simulink model "controlNoLinealModeloCompleto"  (R2023b)
settings: Solver=VariableStepAuto  StartTime=0.0  StopTime=10.0  RelTol=1e-3
values from neighbouring files (symbols this model uses):
  qc = robot.ikine(Tcart,q0,'mask',mask)    [TP_2.m]
libraries: roblocks x8
settings Model: Creator=nmestanza  LastModifiedBy=nmestanza

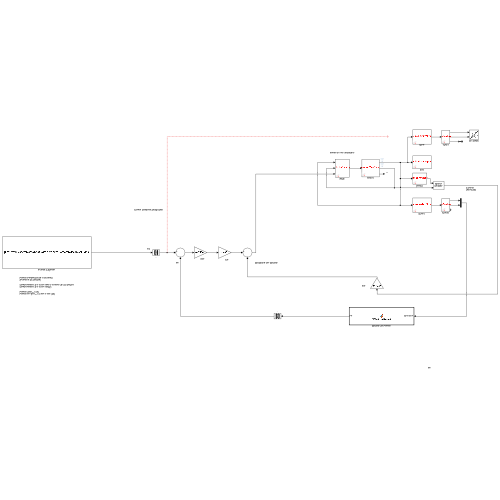
[thumbnail: Simulink's stored preview of the top-level diagram]
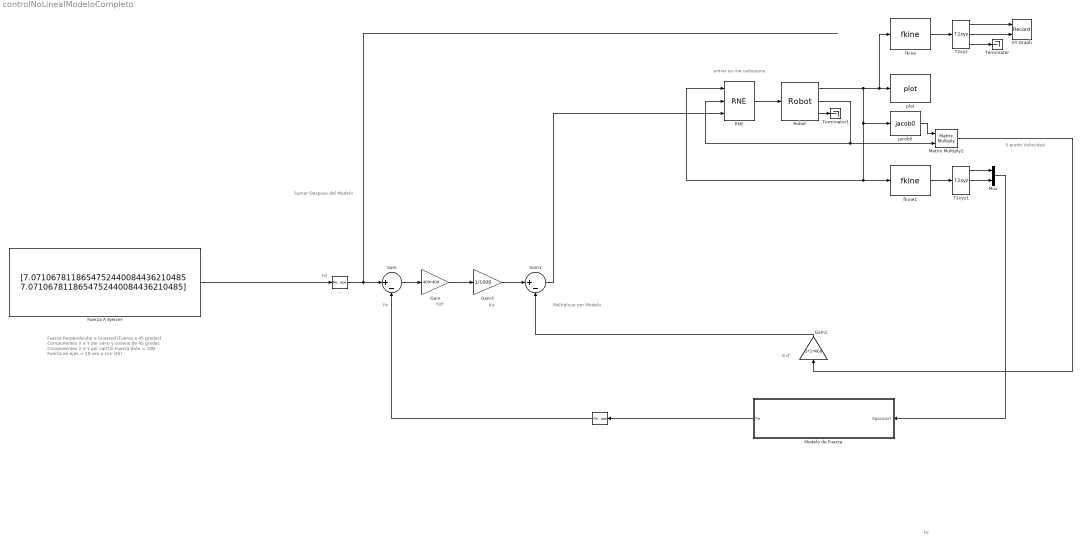
== system controlNoLinealModeloCompleto ==
  note: Multiplicar por Modelo
  note: Sumar Despues del Modelo
  note: X punto
      | Velocidad
  note: Fe
  note: Fe
  note: Kvf
  note: Kpf
  note: Fuerza Perpendicular a la pared
      | (Fuerza a 45 grados)
      |
      | Componentes X e Y por seno y coseno de 45 grados
      | Componentes X e Y por sqrt(2)
      |
      | Fuerza dato = 10N
      | Fuerza en ejes = 10.sen o cos (45)
  note: Ke
  note: Fd
  note: armar un rne cartesiano
  . : Reshape  OutputDimensionality=Column vector (2-D)
  .. : Reshape  OutputDimensionality=Column vector (2-D)
  Fuerza A Ejercer : Constant  Value=[7.0710678118654752440084436210485 7.0710678118654752440084436210485]
  Gain : Gain  Gain=400*400
  Gain1 : Gain  Gain=2*1*400
  Gain3 : Gain  Gain=1/1000
  Matrix Multiply2 : Product  Multiplication=Matrix(*)
  Modelo de Fuerza : MATLAB Function  TreatAsAtomicUnit=on
  Mux : Mux  Inputs=2
  RNE : roblocks/Arm/RNE  robot=robot  grav=[0 0 9.81]
  Robot : roblocks/Arm/Robot  robot=robot  q0=qc(1,:)
  Sum : Sum  Inputs=|+-
  Sum1 : Sum  Inputs=|+-
  T2xyz : roblocks/Toolbox/T2xyz
  T2xyz1 : roblocks/Toolbox/T2xyz
  Terminator : Terminator
  Terminator1 : Terminator
  XY Graph : Record  FileSettingsInternal="{\"entries\":[{\"content\":{\"excelSettings\":{\"content\":{},\"type\":\"Streamout.ExcelSettings\"}},\"type\":\"Streamout.FileSettingStorage\",\"uuid\":\"\"}],\"packageUris\":[\"http:\\/\\/schema.mathworks.com\\/mf0\\/streamout_blocks\\/R2020a\"],\"version\":\"1.0\"}"  Layout=[1 1]  SignalsInternal="{\"entries\":[{\"content\":{\"signals\":[{\"content\":{\"blockPath\":[],\"dimensions\":[1],\"domain\":\"\",\"lineColor\":\"#a2142f\",\"plots\":[1],\"port\":1,\"signalID\":32,\"signalName\":\"XY Graph:1\"},\"type\":\"RecordBlkView.Signal\",\"uuid\":\"\"},{\"content\":{\"blockPath\":[],\"dimensions\":[1],\"domain\":\"\",\"lineColor\":\"#139fff\",\"plots\":[1],\"port\":2,\"signalID\":35,\"signalName\":\"XY Graph:2\"},\"type\":\"RecordBlkView.Signal\",\"uuid\":\"\"}]},\"type\":\"RecordBlkView.InputSignals\",\"uuid\":\"\"}],\"packageUris\":[\"http:\\/\\/schema.mathworks.com\\/mf0\\/streamout_blocks\\/R2020a\"],\"version\":\"1.0\"}"  VisualizationBindings="{\"xyplotplugin\":{\"info\":[{\"series\":[{\"bindingParametersList\":[{\"parameter\":\"X-Axis\",\"signalID\":32,\"signalName\":\"XY Graph:1\"},{\"parameter\":\"Y-Axis\",\"signalID\":35,\"signalName\":\"XY Graph:2\"}],\"seriesID\":44069}],\"subplotID\":1}]}}"  CompatibilityTag=XY  st=-1
  fkine : roblocks/Arm/fkine  robot=robot
  fkine1 : roblocks/Arm/fkine  robot=robot
  "jacob0 " : roblocks/Arm/jacob0   robot=robot
  plot : roblocks/Arm/plot  robot=robot  fps=25  holdplot=off
  wires:
  Modelo de Fuerza/1(Fe) -> ./1
  Fuerza A Ejercer/1 -> ../1
  Gain3/1 -> Sum1/1
  Gain/1 -> Gain3/1
  Sum/1 -> Gain/1
  Gain1/1 -> Sum1/2
  ../1 -> Sum/1
  ./1 -> Sum/2
  T2xyz/1 -> XY Graph/1
  T2xyz/3 -> Terminator/1
  RNE/1 -> Robot/1
  Robot/2 -> RNE/2, Matrix Multiply2/2
  Robot/1 -> fkine/1, plot/1, RNE/1, fkine1/1, "jacob0 "/1
  Robot/3 -> Terminator1/1
  fkine/1 -> T2xyz/1
  "jacob0 "/1 -> Matrix Multiply2/1
  T2xyz/2 -> XY Graph/2
  fkine1/1 -> T2xyz1/1
  T2xyz1/1 -> Mux/1
  T2xyz1/2 -> Mux/2
  Mux/1 -> Modelo de Fuerza/1(Xposicion)
  Matrix Multiply2/1 -> Gain1/1
  Sum1/1 -> RNE/3

== matlab function controlNoLinealModeloCompleto/Modelo de Fuerza ==
  data: Xposicion input; Fe output
%Input: Vector de coordenadas bidimensionales Xposicion como entrada
%Output: Vector de fuerzas bidimensionales Fe 

%Description: Evalar la posición del punto representado por las coordenadas 
%Xposicion con respecto a la pared 
%En base a ello, calcula la fuerza correspondiente.

function Fe = modeloFuerzaCalc(Xposicion)

kEnv = 1000; %N/mm
ejeY = Xposicion(2);
ejeX = Xposicion(1);

%Pared interseca el plano XY en una línea que contiene los puntos (2; 0) y (0; 2)
%Verification Total:
%limY = (ejeX*(-1)+2)/1 = 2 - ejeX
%limX = ((ejeY*1)-2)/-1 = 2 - ejeY
%Por ende:
%ejeX < limX y ejeY< limY
%ejeY < 2 - ejeX ; ejeX < 2 - ejeY
%ejeY + ejeX - 2 + ejeX + ejeY  -2 < 0 
%2ejeX + 2ejeY - 4 < 0 -> ejeX + ejeY - 2 < 0 -> 2 - ejeX - ejeY > 0 fuera
%de pared

%Verifico si el punto está en el lado negativo de la pared
%Calculo la distancia entre el punto y la pared
%Defino la fuerza en función de esa distancia.

if (2-ejeX-ejeY) <= 0 

    distancia = abs(2-ejeX-ejeY)/sqrt(1^2+1^2);
    Fe = [distancia*kEnv*sqrt(2)/2, distancia*kEnv*sqrt(2)/2];

%Verifico si el punto está en el lado positivo de la pared 

else 

    Fe=[0, 0];



end
